simulink model "mcb_pmsm_foc_hall_f28379d"  (R2023b)
settings: Solver=FixedStepDiscrete  StartTime=0.0  StopTime=inf  RelTol=1e-3  EnableMultiTasking=on
InitFcn:
  | mcb_pmsm_foc_hall_f28379d_data;
model workspace (MAT data in the model file):
  encoderResolution = 2000
  hallOffset = '0.5'
  indexOffset = 850
  polePairs = '4'
undefined symbols (not defined in the file): dataType, Down, GPTRIP1SEL, GPTRIP2SEL, inverter, PI_params, pmsm, PosCtrlSpeedLimit, PU_System, target, Ts, Ts_motor, Ts_simulink, Ts_speed, TZ1, TZ2, Up
libraries: simulink x20, c280xlib x17, mcbcontrolslib x9, c2837xDlib x7, c2802xlib x7, svdschedulerlib x5, slpidlib x3, mcbpositiondecoderlib x3, mcbhdlpositiondecoderlib x1, svdutilitieslib x1, mcbplantlib x1, autolibpmsmexterior x1
(part 1 of 4)
settings Model: SimulationMode=external  ExtModeTrigDuration=8  Creator=The MathWorks, Inc.  LastModifiedBy=mdp_3
settings SolverCC: AlgebraicLoopSolver=TrustRegion  AutoInsertRateTranBlk=on
settings DataIOCC: LimitDataPoints=on  SaveFormat=Array  SaveOutput=off  SaveTime=off  ReturnWorkspaceOutputs=off
settings OptimizationCC: DefaultUnderspecifiedDataType=single  OptimizeBlockIOStorage=off  BufferReuse=off  ReuseModelBlockBuffer=off  GlobalBufferReuse=off  ExpressionFolding=off  ExpressionDepthLimit=2147483647  LocalBlockOutputs=off  InitFltsAndDblsToZero=on  NoFixptDivByZeroProtection=on  EfficientFloat2IntCast=on  EfficientMapNaN2IntZero=off  LifeSpan=Inf  MaxStackSize=512  OptimizeDataStoreBuffers=off  BusAssignmentInplaceUpdate=off  EfficientTunableParamExpr=on
settings DebuggingCC: ReadBeforeWriteMsg=DisableAll  WriteAfterWriteMsg=DisableAll  WriteAfterReadMsg=DisableAll  CheckSSInitialOutputMsg=off  SignalResolutionControl=TryResolveAllWithWarning  SolverPrmCheckMsg=warning  InheritedTsInSrcMsg=none  MultiTaskDSMMsg=none  MultiTaskCondExecSysMsg=none  TasksWithSamePriorityMsg=none  SigSpecEnsureSampleTimeMsg=none  IntegerOverflowMsg=none  ParameterPrecisionLossMsg=none  FcnCallInpInsideContextMsg=warning  UnconnectedInputMsg=warning  UnconnectedOutputMsg=warning  UnconnectedLineMsg=warning  AllowSymbolicDim=off  StateNameClashWarn=warning  PregeneratedLibrarySubsystemCodeDiagnostic=none  SFUnexpectedBacktrackingDiag=warning  SFNoUnconditionalDefaultTransitionDiag=warning  SFExecutionAtInitializationDiag=none  IntegerSaturationMsg=none  ArithmeticOperatorsInVariantConditions=warning
settings HardwareCC: ProdBitPerChar=16  ProdBitPerInt=16  ProdBitPerPointer=32  ProdBitPerSizeT=32  ProdBitPerPtrDiffT=32  ProdLargestAtomicInteger=Integer  ProdLargestAtomicFloat=None  ProdWordSize=16  ProdLongLongMode=on  ProdHWDeviceType=Texas Instruments->C2000  TargetBitPerChar=16  TargetBitPerInt=16  TargetBitPerPointer=16  TargetLargestAtomicInteger=Integer  TargetIntDivRoundTo=Zero  TargetEndianess=LittleEndian  TargetWordSize=16  TargetHWDeviceType=TI C2000
settings ModelReferenceCC: EnableRefExpFcnMdlSchedulingChecks=on  PropagateSignalLabelsOutOfModel=off
settings SFSimCC: SimUseLocalCustomCode=off  MATLABDynamicMemAlloc=off
settings SFSimCC: SimCustomHeaderCode=|
  | #include "AHIT_Gimbal_Encoder.h"
  | #include "AHIT_RLS_Encoder_Init.h"
settings SFSimCC: SimUserSources=|
  | AHIT_Gimbal_Encoder.c
  | AHIT_RLS_Encoder_Init.c
settings SFSimCC: SimUserIncludeDirs=|
  | ./include_3
  | ./src_3
settings RTWCC: Description=Embedded Coder  SystemTargetFile=ert.tlc  HardwareBoard=TI Delfino F28379D LaunchPad  TemplateMakefile=ert_default_tmf  GenerateReport=on  RTWUseLocalCustomCode=off  RTWUseSimCustomCode=on  Toolchain=Texas Instruments Code Composer Studio (C2000)  IncludeHyperlinkInReport=on  GenerateTraceInfo=on  GenerateTraceReport=on  GenerateTraceReportSl=on  GenerateTraceReportSf=on  GenerateTraceReportEml=on  DLArmComputeVersion=19.05
settings RTWCC: CustomHeaderCode=|
  | #include "AHIT_Gimbal_Encoder.h"
  | #include "AHIT_RLS_Encoder_Init.h"
settings RTWCC: CustomInclude=|
  | ./include_3
  | ./src_3
settings RTWCC: CustomSource=|
  | AHIT_Gimbal_Encoder.c
  | AHIT_RLS_Encoder_Init.c
settings CodeAppCC: IgnoreCustomStorageClasses=off  CustomSymbolStrType=$N$R$M  StateflowObjectComments=on  InternalIdentifier=Classic
settings ERTTargetCC: CodeReplacementLibrary=TI C28x  MultiwordLength=2048  ConvertIfToSwitch=off  SuppressUnreachableDefaultCases=off  MemSecPackage=tic2000demospkg
settings ConfigComp: CovMetricSettings=dw  CovSaveCumulativeToWorkspaceVar=on  CovSaveSingleToWorkspaceVar=on  CovExternalEMLEnable=off  CovSFcnEnable=off

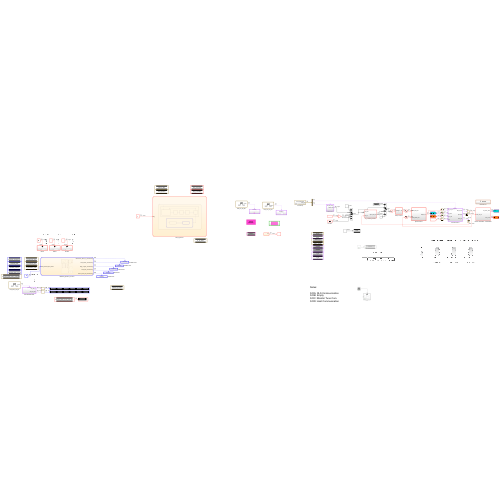
[thumbnail: Simulink's stored preview of the top-level diagram]
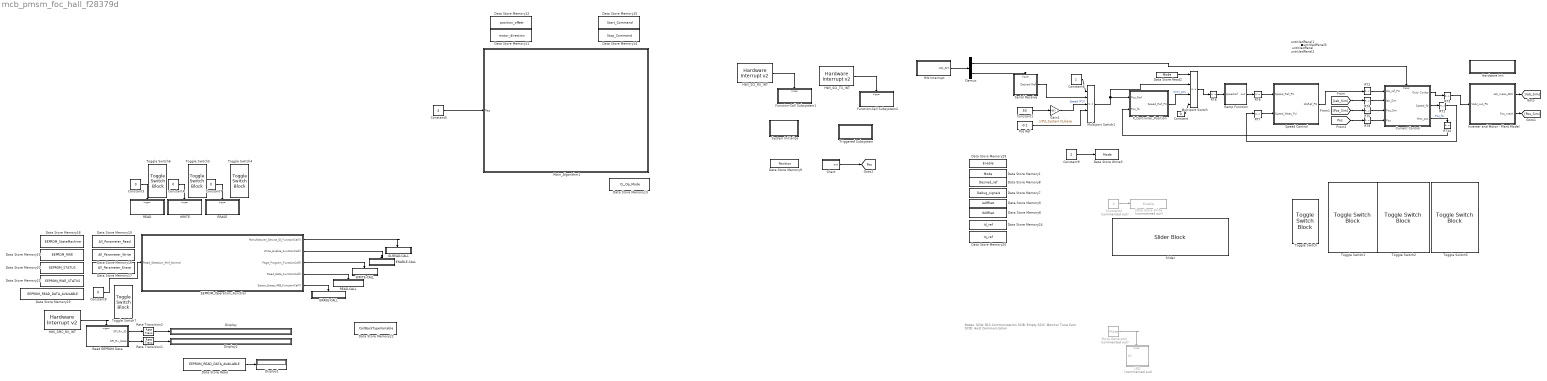
== system mcb_pmsm_foc_hall_f28379d ==
  note: Notes:
      |
      | SCIA: RLS Communication
      | SCIB: Empty
      | SCIC: Monitor Tune Com.
      | SCID: Host Communication
  Chart : Stateflow chart  TreatAsAtomicUnit=on
  Constant : Constant  Value=0  SampleTime=-1
  Constant1 : Constant  Value=50  OutDataTypeStr=single  SampleTime=-1
  Constant2 : Constant  Commented=on  Value=0  OutDataTypeStr=boolean  SampleTime=-1
  Constant3 : Constant  Value=0  OutDataTypeStr=single  SampleTime=-1
  Constant4 : Constant  Value=0  OutDataTypeStr=single  SampleTime=-1
  Constant5 : Constant  Value=4  OutDataTypeStr=uint16  SampleTime=-1
  Constant6 : Constant  SampleTime=-1
  Constant7 : Constant  Value=0  OutDataTypeStr=single  SampleTime=-1
  Constant8 : Constant  Value=0  OutDataTypeStr=boolean  SampleTime=-1
  Constant9 : Constant  Value=2  SampleTime=-1
  Current Control : Subsystem
      settings: RTWSystemCode=Nonreusable function
  Data Store Memory1 : DataStoreMemory  DataStoreName=Mode  ReadBeforeWriteMsg=warning  WriteAfterWriteMsg=warning  WriteAfterReadMsg=warning  InitialValue=500  ShowAdditionalParam=off  OutDataTypeStr=single
  Data Store Memory10 : DataStoreMemory  DataStoreName=All_Parameter_Read  ShowAdditionalParam=off  OutDataTypeStr=boolean
  Data Store Memory11 : DataStoreMemory  DataStoreName=motor_direction  ShowAdditionalParam=off  OutDataTypeStr=uint16
  Data Store Memory12 : DataStoreMemory  DataStoreName=position_offset  ShowAdditionalParam=off  OutDataTypeStr=uint16
  Data Store Memory13 : DataStoreMemory  Description=Closed Loop Operation Mode Selector Variable  DataStoreName=CL_Op_Mode  ShowAdditionalParam=off  OutDataTypeStr=uint16
  Data Store Memory14 : DataStoreMemory  DataStoreName=Stop_Command  ShowAdditionalParam=off  OutDataTypeStr=uint16
  Data Store Memory15 : DataStoreMemory  DataStoreName=Start_Command  ShowAdditionalParam=off  OutDataTypeStr=uint16
  Data Store Memory16 : DataStoreMemory  DataStoreName=All_Parameter_Write  ShowAdditionalParam=off  OutDataTypeStr=boolean
  Data Store Memory17 : DataStoreMemory  DataStoreName=All_Parameter_Erase  ShowAdditionalParam=off  OutDataTypeStr=boolean
  Data Store Memory18 : DataStoreMemory  DataStoreName=EEPROM_StateMachine  InitialValue=t_EEPROM_StateMachine_e.EEPROM_OPERATION_DUMMY_STATE  ShowAdditionalParam=off  OutDataTypeStr=Enum: t_EEPROM_StateMachine_e
  Data Store Memory19 : DataStoreMemory  DataStoreName=EEPROM_RWE  InitialValue=t_EEPROM_RWE_e.EEPROM_DUMMY  ShowAdditionalParam=off  OutDataTypeStr=Enum: t_EEPROM_RWE_e
  Data Store Memory20 : DataStoreMemory  DataStoreName=EEPROM_STATUS  InitialValue=t_EEPROM_STATUS_e.EEPROM_STATUS_NOTBUSY  ShowAdditionalParam=off  OutDataTypeStr=Enum: t_EEPROM_STATUS_e
  Data Store Memory21 : DataStoreMemory  DataStoreName=EEPROM_RWE_STATUS  InitialValue=t_EEPROM_RWE_STATUS_e.EEPROM_RWE_STATUS_DUMMY  ShowAdditionalParam=off  OutDataTypeStr=Enum: t_EEPROM_RWE_STATUS_e
  Data Store Memory22 : DataStoreMemory  DataStoreName=CallBackTypeVariable  ShowAdditionalParam=off  OutDataTypeStr=uint16
  Data Store Memory23 : DataStoreMemory  DataStoreName=EEPROM_READ_DATA_AVAILABLE  ShowAdditionalParam=off  OutDataTypeStr=uint16
  Data Store Memory24 : DataStoreMemory  DataStoreName=Id_ref  ReadBeforeWriteMsg=warning  WriteAfterWriteMsg=warning  WriteAfterReadMsg=warning  ShowAdditionalParam=off  OutDataTypeStr=single
  Data Store Memory25 : DataStoreMemory  DataStoreName=Iq_ref  ReadBeforeWriteMsg=warning  WriteAfterWriteMsg=warning  WriteAfterReadMsg=warning  ShowAdditionalParam=off  OutDataTypeStr=single
  Data Store Memory29 : DataStoreMemory  DataStoreName=Enable  ShowAdditionalParam=off  OutDataTypeStr=boolean
  Data Store Memory5 : DataStoreMemory  DataStoreName=IaOffset  InitialValue=inverter.CtSensAOffset  ShowAdditionalParam=off
  Data Store Memory6 : DataStoreMemory  DataStoreName=IbOffset  InitialValue=inverter.CtSensBOffset  ShowAdditionalParam=off
  Data Store Memory7 : DataStoreMemory  DataStoreName=Debug_signals  ReadBeforeWriteMsg=warning  WriteAfterWriteMsg=warning  WriteAfterReadMsg=warning  InitialValue=5  ShowAdditionalParam=off  OutDataTypeStr=uint16
  Data Store Memory8 : DataStoreMemory  DataStoreName=Desired_ref  ReadBeforeWriteMsg=warning  WriteAfterWriteMsg=warning  WriteAfterReadMsg=warning  InitialValue=500  ShowAdditionalParam=off  OutDataTypeStr=dataType
  Data Store Memory9 : DataStoreMemory  DataStoreName=Position  WriteAfterWriteMsg=warning  ShowAdditionalParam=off  OutDataTypeStr=single
  Data Store Read : DataStoreRead  DataStoreName=EEPROM_READ_DATA_AVAILABLE  IndexOptions=Index vector (dialog)  Indices=1  OutputSizes=1
  Data Store Write : DataStoreWrite  Commented=on  DataStoreName=Enable  IndexOptions=Index vector (dialog)  Indices=1  OutputSizes=1
  Data Store Write3 : DataStoreWrite  DataStoreName=Mode  IndexOptions=Index vector (dialog)  Indices=1  OutputSizes=1
  Data Store Read2 : DataStoreRead  DataStoreName=Mode  IndexOptions=Index vector (dialog)  Indices=1  OutputSizes=1
  Demux : Demux  Outputs=2
  Display : Display
      settings: Format=hex (Stored Integer)
  Display1 : Display
  Display2 : Display
      settings: Format=hex (Stored Integer)
  EEPROM_Operation_Function : Stateflow chart  TreatAsAtomicUnit=on  SystemSampleTime=1/10
  ENABLE-CALL : Subsystem  TreatAsAtomicUnit=on
  ERASE : Subsystem  TreatAsAtomicUnit=on
  ERASE-CALL : Subsystem  TreatAsAtomicUnit=on
  Function-Call Subsystem1 : Subsystem  TreatAsAtomicUnit=on
  Function-Call Subsystem2 : Subsystem  TreatAsAtomicUnit=on
  Gain1 : Gain  Gain=1/PU_System.N_base  RndMeth=Simplest  OutDataTypeStr=Inherit: Same as input
  HW Interrupt : Subsystem  Variant=on  VariantControlMode=sim codegen switching
  HWI_SCI_RX_INT : svdschedulerlib/Hardware Interrupt v2  ISRGroup=ADC - Analog to Digital Converter  ISRName=ADCA1_INT  ISRNumber=32  NumEventsToServe=1  EventsList={'on','EOC event','1';'off','Overflow event','2';'off','Custom event','3'}  SelectedEvents={'event1'}  TaskPriority=25  DisablePreemption=off  ClearInterruptFlagsAtEndOfEvent=on  InterruptDefinitionFile=$(TARGET_ROOT)/registry/interrupts/F2837xS_interrupts.xml  HardwareBoard=F2837x  EnableSimPort=off
      settings: LibrarySourceBlock=c2000lib/Scheduling/Hardware Interrupt
  HWI_SCI_TX_INT : svdschedulerlib/Hardware Interrupt v2  ISRGroup=ADC - Analog to Digital Converter  ISRName=ADCA1_INT  ISRNumber=32  NumEventsToServe=1  EventsList={'on','EOC event','1';'off','Overflow event','2';'off','Custom event','3'}  SelectedEvents={'event1'}  TaskPriority=25  DisablePreemption=off  ClearInterruptFlagsAtEndOfEvent=on  InterruptDefinitionFile=$(TARGET_ROOT)/registry/interrupts/F2837xS_interrupts.xml  HardwareBoard=F2837x  EnableSimPort=off
      settings: LibrarySourceBlock=c2000lib/Scheduling/Hardware Interrupt
  HWI_SPIC_RX_INT : svdschedulerlib/Hardware Interrupt v2  ISRGroup=ADC - Analog to Digital Converter  ISRName=ADCA1_INT  ISRNumber=32  NumEventsToServe=1  EventsList={'on','EOC event','1';'off','Overflow event','2';'off','Custom event','3'}  SelectedEvents={'event1'}  TaskPriority=50  DisablePreemption=off  ClearInterruptFlagsAtEndOfEvent=on  InterruptDefinitionFile=$(TARGET_ROOT)/registry/interrupts/F2837xS_interrupts.xml  HardwareBoard=F2837x  EnableSimPort=off
      settings: LibrarySourceBlock=c2000lib/Scheduling/Hardware Interrupt
  Hardware Init : Subsystem  TreatAsAtomicUnit=on
  ID-READ-CALL : Subsystem  TreatAsAtomicUnit=on
  Inverter and Motor - Plant Model : Subsystem
  LED : Subsystem  Commented=on
  Main_Algorithm1 : Stateflow chart  TreatAsAtomicUnit=on
  Multiport Switch : MultiPortSwitch  Inputs=2  DataPortForDefault=Additional data port  SaturateOnIntegerOverflow=off  InputSameDT=off
  Multiport Switch1 : MultiPortSwitch  DataPortForDefault=Additional data port  SaturateOnIntegerOverflow=off  InputSameDT=off
  P_Controller_Position : Subsystem
  Pos Ref : Constant  Value=-0.1  OutDataTypeStr=single  SampleTime=-1
  Pulse Generator : DiscretePulseGenerator  Commented=on  PulseType=Time based  Period=0.5  PulseWidth=50
  READ : Subsystem  TreatAsAtomicUnit=on
  READ-CALL : Subsystem  TreatAsAtomicUnit=on
  RT{1,6..8,10} (5 alike) : RateTransition  Deterministic=off  OutPortSampleTime=Ts_speed
  RT{2..5,9} (5 alike) : RateTransition  Deterministic=off
  Ramp Function : Subsystem  TreatAsAtomicUnit=on  SystemSampleTime=Ts_speed
  Rate Transition1 : RateTransition  Deterministic=off  OutPortSampleTime=0.2
  Rate Transition2 : RateTransition  Deterministic=off  OutPortSampleTime=0.2
  Read EEPROM Data : Subsystem
  Serial Receive : Subsystem  SystemSampleTime=1e-3
  Slider : SliderBlock  ScaleMax=300
  Speed Control : Subsystem  TreatAsAtomicUnit=on  SystemSampleTime=Ts_speed
  System Initialize : Subsystem  mask(System Initialize){ShowInLibBrowser=0}
      mask prompts: ShowInLibBrowser "Simulink:masks:CustCodeMaskParam1_MP"
      settings: CopyFcn=cccopyfcn(gcb)  OpenFcn=ccopenfcn('System Initialize Function')
      mask Help: eval('feval(''rtwprivate'',''rtwhelpview'',''rtw_sys_initialize_block'')');
      mask Display: disp('System\nInitialize');
  Toggle Switch{,4..7} (5 alike) : ToggleSwitchBlock
      settings: Values={{'Off', 'On'}, [0 1]}
  Toggle Switch1 : ToggleSwitchBlock  LabelPosition=Bottom
      settings: Values={{'Manual Speed Param En', 'Calculated Speed Param En'}, [0 1]}
  Toggle Switch2 : ToggleSwitchBlock  LabelPosition=Bottom
      settings: Values={{'Manual D Loop Param En', 'Calculated D Loop Param En'}, [0 1]}
  Toggle Switch3 : ToggleSwitchBlock  LabelPosition=Bottom
      settings: Values={{'Manual Q Loop Param En', 'Calculated Q Loop Param En'}, [0 1]}
  Triggered Subsystem : Subsystem  TreatAsAtomicUnit=on  SystemSampleTime=0.01
  WRITE : Subsystem  TreatAsAtomicUnit=on
  WRITE-CALL : Subsystem  TreatAsAtomicUnit=on
  untitledPanel : Subsystem  Tag=HiddenForWebPanel  IsWebBlockPanel=on
  untitledPanel1 : Subsystem  Tag=HiddenForWebPanel  IsWebBlockPanel=on
  untitledPanel2 : Subsystem  Tag=HiddenForWebPanel  IsWebBlockPanel=on
  untitledPanel3 : Subsystem  Tag=HiddenForWebPanel  IsWebBlockPanel=on
  tag scope: Pos=global
  wires:
  RT1/1 -> RT7/1
  [Iab_Sim] -> RT4/1
  Speed Control/1(IdqRef_PU) -> RT2/1
  [Pos_Sim] -> RT5/1
  RT2/1 -> Current Control/1(Idq_ref_PU)
  RT4/1 -> Current Control/2(Iab_Sim)
  RT5/1 -> Current Control/3(Pos_Sim)
  Current Control/1(Duty Cycles) -> RT3/1
  RT3/1 -> Inverter and Motor - Plant Model/1(Vabc_out_PU)
  Inverter and Motor - Plant Model/1(Iab_meas_ADC) -> [Iab_Sim]
  Inverter and Motor - Plant Model/2(Pos_mech) -> [Pos_Sim]
  Current Control/2(Speed_fb) -> RT1/1
  Demux/2 -> Serial Receive/Trigger
  Demux/1 -> Current Control/Trigger
  HW Interrupt/1(HW_INT) -> Demux/1
  RT6/1 -> Speed Control/1(Speed_Ref_PU)
  RT7/1 -> Speed Control/2(Speed_Meas_PU)
  RT8/1 -> Ramp Function/1(speedref)
  Ramp Function/1(out) -> RT6/1
  Constant1/1 -> Gain1/1
  Constant2/1 -> Data Store Write/1
  Pulse Generator/1 -> LED/Trigger
  HWI_SCI_TX_INT/1 -> Function-Call Subsystem2/Trigger
  HWI_SCI_RX_INT/1 -> Function-Call Subsystem1/Trigger
  [Pos] -> RT9/1
  RT9/1 -> Current Control/4(Pos)
  EEPROM_Operation_Function/2(Write_Enable_FunctionCall()) -> ENABLE-CALL/Trigger
  Constant7/1 -> ERASE/Trigger
  Rate Transition1/1 -> Display2/1
  Rate Transition2/1 -> Display/1
  Read EEPROM Data/1(SPI_Rx_ID) -> Rate Transition2/1
  EEPROM_Operation_Function/3(Page_Program_FunctionCall()) -> WRITE-CALL/Trigger
  EEPROM_Operation_Function/5(Sector_Erase_4KB_FunctionCall()) -> ERASE-CALL/Trigger
  Read EEPROM Data/2(SPI_Rx_Data) -> Rate Transition1/1
  EEPROM_Operation_Function/4(Read_Data_FunctionCall()) -> READ-CALL/Trigger
  Constant3/1 -> READ/Trigger
  Constant8/1 -> EEPROM_Operation_Function/1(Read_Selection_Mnf_Normal)
  HWI_SPIC_RX_INT/1 -> Read EEPROM Data/Trigger
  Constant4/1 -> WRITE/Trigger
  EEPROM_Operation_Function/1(Manufacturer_Device_ID_FunctionCall()) -> ID-READ-CALL/Trigger
  Data Store Read/1 -> Display1/1
  Chart/1(out) -> [Pos]
  Constant5/1 -> Main_Algorithm1/1(flag)
  Current Control/3(Mec_pos) -> RT10/1  "Pos_fb"
  RT10/1 -> P_Controller_Position/2(Pos_fb)
  Data Store Read2/1 -> Multiport Switch/1
  P_Controller_Position/1(Speed_Ref_PU) -> Multiport Switch/3  "error_pos"
  Multiport Switch/1 -> RT8/1
  Constant/1 -> Multiport Switch/4
  Multiport Switch1/1 -> Multiport Switch/2, P_Controller_Position/1(Pos_Ref)
  Serial Receive/1(Desired Ref) -> Multiport Switch1/2
  Constant6/1 -> Multiport Switch1/1
  Gain1/1 -> Multiport Switch1/3  "Speed (PU)"
  Pos Ref/1 -> Multiport Switch1/4
  Constant9/1 -> Data Store Write3/1

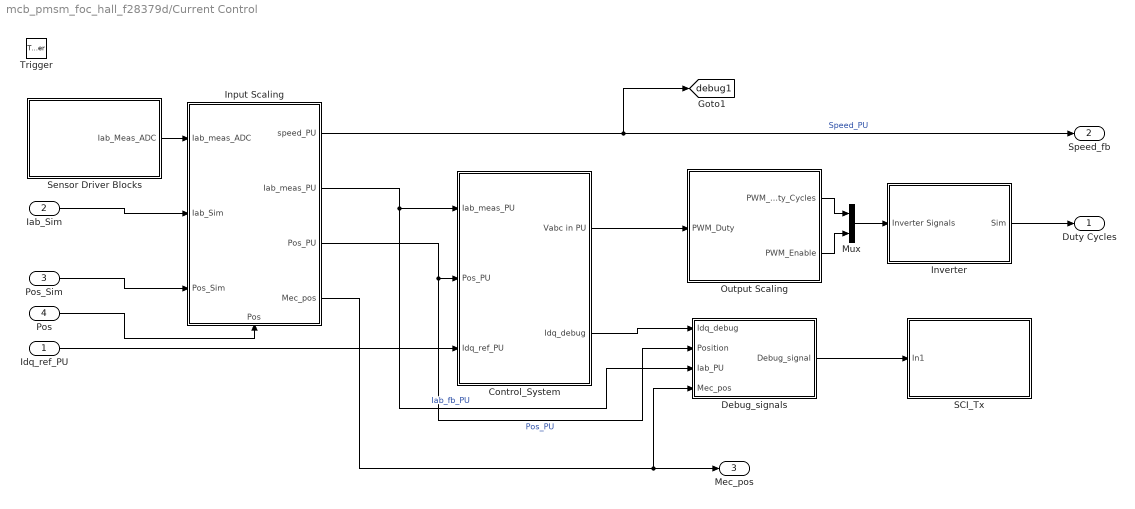
== system mcb_pmsm_foc_hall_f28379d/Current Control ==
  Idq_ref_PU : Inport
  Iab_Sim : Inport  Port=2
  Pos_Sim : Inport  Port=3
  Pos : Inport  Port=4
  Trigger : TriggerPort  TriggerType=function-call  VariantControl=Variant  PortDimensions=1
  Control_System : Subsystem
  Debug_signals : Subsystem
  Input Scaling : Subsystem  Variant=on  VariantControlMode=sim codegen switching  VariantControl=Variant1  PropagateVariantConditions=on
      settings: PortSchema="{\"entries\":[{\"content\":{\"sides\":[{\"content\":{\"connectorIds\":[\"In1\",\"In2\",\"In3\"]},\"type\":\"ConnectorPlacement.EquallySpacedRectSide\",\"uuid\":\"9f2f3667-6d5e-4714-8728-a7ac227716ab\"},{\"content\":{\"connectorIds\":[\"Out1\",\"Out2\",\"Out3\",\"Out4\"],\"side\":\"RIGHT\"},\"type\":\"ConnectorPlacement.EquallySpacedRectSide\",\"uuid\":\"67095e94-5e6f-40af-88f8-fd5db9288dde\"},{\"content\":{\"side\":\"TOP\"},\"type\":\"ConnectorPlacement.EquallySpacedRectSide\",\"uuid\":\"f24a6960-aaac-4f51-bbf1-cf742b655049\"},{\"content\":{\"connectorIds\":[\"In4\"],\"side\":\"BOTTOM\"},\"type\":\"ConnectorPlacement.EquallySpacedRectSide\",\"uuid\":\"f0da2b81-93a9-4692-bf57-8dbb868edb44\"}]},\"type\":\"ConnectorPlacement.EquallySpacedConnector\",\"uuid\":\"0556ef15-0a97-49bd-aca6-6a1187ae6596\"}],\"packageUris\":[\"http://schema.mathworks.com/mf0/Connector/R2020b\"],\"version\":\"1.0\"}"
  Inverter : Subsystem  Variant=on  VariantControlMode=sim codegen switching
  Mux : Mux  Inputs=2
  Output Scaling : Subsystem
  SCI_Tx : Subsystem  Variant=on  VariantControlMode=sim codegen switching
  Sensor Driver Blocks : Subsystem  Variant=on  VariantControlMode=sim codegen switching
  Duty Cycles : Outport  InitialOutput=0  VectorParamsAs1DForOutWhenUnconnected=off
  Speed_fb : Outport  Port=2  InitialOutput=0  VectorParamsAs1DForOutWhenUnconnected=off
  Mec_pos : Outport  Port=3  InitialOutput=0  VectorParamsAs1DForOutWhenUnconnected=off
  tag scope: debug1=global
  wires:
  Control_System/1(Vabc in PU) -> Output Scaling/1(PWM_Duty)
  Input Scaling/3(Pos_PU) -> Debug_signals/2(Position), Control_System/2(Pos_PU)  "Pos_PU"
  Idq_ref_PU/1 -> Control_System/3(Idq_ref_PU)
  Input Scaling/1(speed_PU) -> [debug1], Speed_fb/1  "Speed_PU"
  Input Scaling/2(Iab_meas_PU) -> Debug_signals/3(Iab_PU), Control_System/1(Iab_meas_PU)  "Iab_fb_PU"
  Sensor Driver Blocks/1(Iab_Meas_ADC) -> Input Scaling/1(Iab_meas_ADC)
  Iab_Sim/1 -> Input Scaling/2(Iab_Sim)
  Pos_Sim/1 -> Input Scaling/3(Pos_Sim)
  Inverter/1(Sim) -> Duty Cycles/1
  Debug_signals/1(Debug_signal) -> SCI_Tx/1(In1)
  Mux/1 -> Inverter/1(Inverter Signals)
  Output Scaling/2(PWM_Enable) -> Mux/2
  Output Scaling/1(PWM_Duty_Cycles) -> Mux/1
  Control_System/2(Idq_debug) -> Debug_signals/1(Idq_debug)
  Pos/1 -> Input Scaling/4(Pos)
  Input Scaling/4(Mec_pos) -> Debug_signals/4(Mec_pos), Mec_pos/1

== system mcb_pmsm_foc_hall_f28379d/ENABLE-CALL ==
  function : TriggerPort  TriggerType=function-call  VariantControl=(inherit)
  Chart : Stateflow chart  Commented=on  TreatAsAtomicUnit=on
  Data Store Write1 : DataStoreWrite  DataStoreName=CallBackTypeVariable  IndexOptions=Index vector (dialog)  Indices=1  OutputSizes=1
  Read Command : Constant  Value=6  OutDataTypeStr=uint16  SampleTime=-1
  SPI Transmit : c280xlib/SPI Transmit  Priority=1  SPISelect=SPI_C  ClockPolarity=Rising_edge  ClockPhase=Delay_half_cycle  SPIModule=uint32(0)  Mode=Master  BusSpeed=uint32(1000000)  FirstBitToTransfer=Most significant bit (MSB)  ClockMode=0  BlockFunction=Write  EnableRegisterAddress=on  RegisterAddress=0  OutputDataType=int8  OutputDataLength=1  BlockingMode=on  DataBits=8  UseCustomSSPin=Explicit GPIO calls  ActiveLowSSPin=Active low  Pin=49
  Scope : Scope  Commented=on
  commad : Constant  Value=2  OutDataTypeStr=uint16  SampleTime=-1
  wires:
  Chart/1(output) -> Scope/1
  commad/1 -> Data Store Write1/1
  Read Command/1 -> SPI Transmit/1

== system mcb_pmsm_foc_hall_f28379d/ERASE ==
  Trigger : TriggerPort  VariantControl=(inherit)
  Constant : Constant  OutDataTypeStr=boolean  SampleTime=-1
  Data Store Write2 : DataStoreWrite  DataStoreName=All_Parameter_Erase  IndexOptions=Index vector (dialog)  Indices=1  OutputSizes=1
  wires:
  Constant/1 -> Data Store Write2/1

== system mcb_pmsm_foc_hall_f28379d/ERASE-CALL ==
  function : TriggerPort  TriggerType=function-call  VariantControl=(inherit)
  Chart : Stateflow chart  Commented=on  TreatAsAtomicUnit=on
  Constant : Constant  Value=zeros(3,1)  OutDataTypeStr=uint16  SampleTime=-1
  Data Store Write1 : DataStoreWrite  DataStoreName=CallBackTypeVariable  IndexOptions=Index vector (dialog)  Indices=1  OutputSizes=1
  Mux : Mux  Inputs=2
  Read Command : Constant  Value=32  OutDataTypeStr=uint16  SampleTime=-1
  SPI Transmit : c280xlib/SPI Transmit  Priority=1  SPISelect=SPI_C  ClockPolarity=Rising_edge  ClockPhase=Delay_half_cycle  SPIModule=uint32(0)  Mode=Master  BusSpeed=uint32(1000000)  FirstBitToTransfer=Most significant bit (MSB)  ClockMode=0  BlockFunction=Write  EnableRegisterAddress=on  RegisterAddress=0  OutputDataType=int8  OutputDataLength=1  BlockingMode=on  DataBits=8  UseCustomSSPin=Explicit GPIO calls  ActiveLowSSPin=Active low  Pin=49
  Scope : Scope  Commented=on
  commad : Constant  Value=5  OutDataTypeStr=uint16  SampleTime=-1
  wires:
  Chart/1(output) -> Scope/1
  commad/1 -> Data Store Write1/1
  Constant/1 -> Mux/2  "SPI_Tx_Dummy1"
  Read Command/1 -> Mux/1
  Mux/1 -> SPI Transmit/1  "TX_DATA"

== system mcb_pmsm_foc_hall_f28379d/Function-Call Subsystem1 ==
  function : TriggerPort  TriggerType=function-call  VariantControl=(inherit)
  Data Type Conversion : DataTypeConversion  OutDataTypeStr=uint16  SaturateOnIntegerOverflow=off  RndMeth=Floor
  SCI Receive : c280xlib/SCI Receive  Priority=2  sciModule=A  dataHead=''  headerCheckMaxCount=0  dataTail=''  dataType=uint8  dataLenOptions=Length via dialog  dataDim=1  maxDataLength=1  initValue=0  errOption=Output the last received value  errValue=0  sampleTime=-1  blockingMode=off  timeOut=inf  outputStatus=off
      settings: LibrarySourceBlock=c2837xDlib/SCI Receive
  System Update : Subsystem  mask(System Update){ShowInLibBrowser=0}
      mask prompts: ShowInLibBrowser "Simulink:masks:CustCodeMaskParam1_MP"
      settings: CopyFcn=cccopyfcn(gcb)  OpenFcn=ccopenfcn('System Update Function')
      mask Help: eval('feval(''rtwprivate'',''rtwhelpview'',''rtw_sys_update_block'')');
      mask Display: disp('System\nUpdate');
  Terminator : Terminator
  wires:
  SCI Receive/1 -> Data Type Conversion/1
  Data Type Conversion/1 -> Terminator/1

== system mcb_pmsm_foc_hall_f28379d/Function-Call Subsystem2 ==
  function : TriggerPort  TriggerType=function-call  VariantControl=(inherit)
  SCI Transmit : c280xlib/SCI Transmit  sciModule=A  dataHead=''  dataTail=''  frameSize=1  blockingMode=off  outputStatus=off
      settings: LibrarySourceBlock=c2837xDlib/SCI Transmit

== system mcb_pmsm_foc_hall_f28379d/HW Interrupt ==
  Code Generation : Subsystem  VariantControl=(codegen)
  Simulation : Subsystem  VariantControl=(sim)
  HW_INT : Outport  VectorParamsAs1DForOutWhenUnconnected=off  OutputFunctionCall=on

== system mcb_pmsm_foc_hall_f28379d/Hardware Init ==
  note: Power UP Regulator
  6PWM_Mode : Constant  Priority=1000  Commented=on  Value=0x3A16  OutDataTypeStr=uint16  SampleTime=-1
  ADC_Gain_Setting : Constant  Priority=1000  Commented=on  Value=inverter.SPI_Gain_Setting  OutDataTypeStr=uint16  SampleTime=-1
  Constant : Constant  OutDataTypeStr=boolean  SampleTime=-1
  Constant1 : Constant  OutDataTypeStr=boolean  SampleTime=-1
  Constant2 : Constant  OutDataTypeStr=boolean  SampleTime=-1
  Digital Output : c2837xDlib/Digital Output  GPIO_Number=GPIO144~GPIO151  GPIO_Bit0=off  GPIO_BIT0_Toggle=off  GPIO_Bit1=on  GPIO_BIT1_Toggle=off  GPIO_Bit2=off  GPIO_BIT2_Toggle=off  GPIO_Bit3=off  GPIO_BIT3_Toggle=off  GPIO_Bit4=off  GPIO_BIT4_Toggle=off  GPIO_Bit5=off  GPIO_BIT5_Toggle=off  GPIO_Bit6=off  GPIO_BIT6_Toggle=off  GPIO_Bit7=off  GPIO_BIT7_Toggle=off
  Digital Output1 : c2837xDlib/Digital Output  GPIO_Number=GPIO144~GPIO151  GPIO_Bit0=off  GPIO_BIT0_Toggle=off  GPIO_Bit1=off  GPIO_BIT1_Toggle=off  GPIO_Bit2=on  GPIO_BIT2_Toggle=off  GPIO_Bit3=off  GPIO_BIT3_Toggle=off  GPIO_Bit4=off  GPIO_BIT4_Toggle=off  GPIO_Bit5=off  GPIO_BIT5_Toggle=off  GPIO_Bit6=off  GPIO_BIT6_Toggle=off  GPIO_Bit7=off  GPIO_BIT7_Toggle=off
  Digital Output2 : c2837xDlib/Digital Output  GPIO_Number=GPIO144~GPIO151  GPIO_Bit0=off  GPIO_BIT0_Toggle=off  GPIO_Bit1=off  GPIO_BIT1_Toggle=off  GPIO_Bit2=off  GPIO_BIT2_Toggle=off  GPIO_Bit3=on  GPIO_BIT3_Toggle=off  GPIO_Bit4=off  GPIO_BIT4_Toggle=off  GPIO_Bit5=off  GPIO_BIT5_Toggle=off  GPIO_Bit6=off  GPIO_BIT6_Toggle=off  GPIO_Bit7=off  GPIO_BIT7_Toggle=off
  Event Listener : EventListener  DisableCoverage=on  EventName=reset
  Mux : Mux  Commented=on  Inputs=2
  Variant Subsystem : Subsystem  Commented=on  Variant=on  VariantControlMode=sim codegen switching
  wires:
  6PWM_Mode/1 -> Mux/1
  ADC_Gain_Setting/1 -> Mux/2
  Mux/1 -> Variant Subsystem/1(In1)
  Constant/1 -> Digital Output/1
  Constant1/1 -> Digital Output1/1
  Constant2/1 -> Digital Output2/1

== system mcb_pmsm_foc_hall_f28379d/ID-READ-CALL ==
  function : TriggerPort  TriggerType=function-call  VariantControl=(inherit)
  Chart : Stateflow chart  Commented=on  TreatAsAtomicUnit=on
  Constant : Constant  Value=zeros(3,1)  OutDataTypeStr=uint16  SampleTime=-1
  Data Store Write1 : DataStoreWrite  DataStoreName=CallBackTypeVariable  IndexOptions=Index vector (dialog)  Indices=1  OutputSizes=1
  Mux : Mux  Inputs=3
  Read Address : Constant  Value=[0 0]  OutDataTypeStr=uint16  SampleTime=-1
  Read Command : Constant  Value=144  OutDataTypeStr=uint16  SampleTime=-1
  SPI Transmit : c280xlib/SPI Transmit  Priority=1  SPISelect=SPI_C  ClockPolarity=Rising_edge  ClockPhase=Delay_half_cycle  SPIModule=uint32(0)  Mode=Master  BusSpeed=uint32(1000000)  FirstBitToTransfer=Most significant bit (MSB)  ClockMode=0  BlockFunction=Write  EnableRegisterAddress=on  RegisterAddress=0  OutputDataType=int8  OutputDataLength=1  BlockingMode=on  DataBits=8  UseCustomSSPin=Explicit GPIO calls  ActiveLowSSPin=Active low  Pin=49
  Scope : Scope  Commented=on
  commad : Constant  OutDataTypeStr=uint16  SampleTime=-1
  wires:
  Chart/1(output) -> Scope/1
  Read Address/1 -> Mux/2
  Read Command/1 -> Mux/1
  Constant/1 -> Mux/3  "SPI_Tx_Dummy1"
  Mux/1 -> SPI Transmit/1  "TX_DATA"
  commad/1 -> Data Store Write1/1

== system mcb_pmsm_foc_hall_f28379d/Inverter and Motor - Plant Model ==
  Vabc_out_PU : Inport
  Codegeneration : Subsystem
  Simulation : Subsystem
  Variant Sink : VariantSink  VariantControlMode=sim codegen switching
  Variant Source : VariantSource  VariantControlMode=sim codegen switching
  Variant Source1 : VariantSource  VariantControlMode=sim codegen switching
  Iab_meas_ADC : Outport  VectorParamsAs1DForOutWhenUnconnected=off
  Pos_mech : Outport  Port=2  VectorParamsAs1DForOutWhenUnconnected=off
  wires:
  Codegeneration/2(Pos_fb_Sim) -> Variant Source1/1
  Codegeneration/1(Iab_fb_Sim) -> Variant Source/1
  Variant Source1/1 -> Pos_mech/1
  Variant Sink/1 -> Codegeneration/1(Duty_Cycles)
  Variant Source/1 -> Iab_meas_ADC/1
  Simulation/1(Iab_fb_Sim) -> Variant Source/2
  Variant Sink/2 -> Simulation/1(Duty_Cycles)
  Simulation/2(Pos_fb_Sim) -> Variant Source1/2
  Vabc_out_PU/1 -> Variant Sink/1

== system mcb_pmsm_foc_hall_f28379d/LED ==
  In1 : Inport
  Trigger : TriggerPort  VariantControl=(inherit)  PortDimensions=1
  Constant : Constant  OutDataTypeStr=boolean
  Constant1 : Constant  OutDataTypeStr=boolean
  Digital Output : c2837xDlib/Digital Output  GPIO_Number=GPIO120~GPIO127  GPIO_Bit0=off  GPIO_BIT0_Toggle=off  GPIO_Bit1=off  GPIO_BIT1_Toggle=off  GPIO_Bit2=off  GPIO_BIT2_Toggle=off  GPIO_Bit3=off  GPIO_BIT3_Toggle=off  GPIO_Bit4=off  GPIO_BIT4_Toggle=off  GPIO_Bit5=off  GPIO_BIT5_Toggle=off  GPIO_Bit6=off  GPIO_BIT6_Toggle=off  GPIO_Bit7=on  GPIO_BIT7_Toggle=on
  Digital Output1 : c2837xDlib/Digital Output  GPIO_Number=GPIO128~GPIO135  GPIO_Bit0=on  GPIO_BIT0_Toggle=on  GPIO_Bit1=off  GPIO_BIT1_Toggle=off  GPIO_Bit2=off  GPIO_BIT2_Toggle=off  GPIO_Bit3=off  GPIO_BIT3_Toggle=off  GPIO_Bit4=off  GPIO_BIT4_Toggle=off  GPIO_Bit5=off  GPIO_BIT5_Toggle=off  GPIO_Bit6=off  GPIO_BIT6_Toggle=off  GPIO_Bit7=off  GPIO_BIT7_Toggle=off
  wires:
  Constant1/1 -> Digital Output1/1
  Constant/1 -> Digital Output/1

== system mcb_pmsm_foc_hall_f28379d/P_Controller_Position ==
  Pos_Ref : Inport
  Pos_fb : Inport  Port=2
  Constant : Constant  Value=0.01  OutDataTypeStr=dataType  SampleTime=-1
  Divide : Product  Inputs=**  OutDataTypeStr=dataType  RndMeth=Simplest
  Saturation : Saturate  UpperLimit=PosCtrlSpeedLimit  LowerLimit=-PosCtrlSpeedLimit
  Sum : Sum  Inputs=|+-  OutDataTypeStr=Inherit: Same as first input
  Speed_Ref_PU : Outport
  wires:
  Constant/1 -> Divide/2
  Saturation/1 -> Speed_Ref_PU/1
  Divide/1 -> Saturation/1
  Pos_Ref/1 -> Sum/1
  Pos_fb/1 -> Sum/2
  Sum/1 -> Divide/1

== system mcb_pmsm_foc_hall_f28379d/READ ==
  Trigger : TriggerPort  VariantControl=(inherit)
  Constant : Constant  OutDataTypeStr=boolean  SampleTime=-1
  Data Store Write1 : DataStoreWrite  DataStoreName=All_Parameter_Read  IndexOptions=Index vector (dialog)  Indices=1  OutputSizes=1
  wires:
  Constant/1 -> Data Store Write1/1

== system mcb_pmsm_foc_hall_f28379d/READ-CALL ==
  function : TriggerPort  TriggerType=function-call  VariantControl=(inherit)
  Chart : Stateflow chart  Commented=on  TreatAsAtomicUnit=on
  Constant : Constant  Value=[0 0]  OutDataTypeStr=uint16  SampleTime=-1
  Data Store Write1 : DataStoreWrite  DataStoreName=CallBackTypeVariable  IndexOptions=Index vector (dialog)  Indices=1  OutputSizes=1
  Mux : Mux  Inputs=3
  Read Address : Constant  Value=[0 0 0]  OutDataTypeStr=uint16  SampleTime=-1
  Read Command : Constant  Value=3  OutDataTypeStr=uint16  SampleTime=-1
  SPI Transmit : c280xlib/SPI Transmit  Priority=1  SPISelect=SPI_C  ClockPolarity=Rising_edge  ClockPhase=Delay_half_cycle  SPIModule=uint32(0)  Mode=Master  BusSpeed=uint32(1000000)  FirstBitToTransfer=Most significant bit (MSB)  ClockMode=0  BlockFunction=Write  EnableRegisterAddress=on  RegisterAddress=0  OutputDataType=int8  OutputDataLength=1  BlockingMode=on  DataBits=8  UseCustomSSPin=Explicit GPIO calls  ActiveLowSSPin=Active low  Pin=49
  Scope : Scope  Commented=on
  commad : Constant  Value=4  OutDataTypeStr=uint16  SampleTime=-1
  wires:
  Chart/1(output) -> Scope/1
  commad/1 -> Data Store Write1/1
  Mux/1 -> SPI Transmit/1  "TX_DATA"
  Read Address/1 -> Mux/2
  Constant/1 -> Mux/3  "SPI_Tx_Dummy1"
  Read Command/1 -> Mux/1

== system mcb_pmsm_foc_hall_f28379d/Ramp Function ==
  speedref : Inport
  Chart : Stateflow chart  TreatAsAtomicUnit=on
  Constant : Constant  Value=0.1  OutDataTypeStr=single  SampleTime=-1
  Constant1 : Constant  Value=0.1  OutDataTypeStr=single  SampleTime=-1
  Constant2 : Constant  Value=Ts_speed  OutDataTypeStr=single  SampleTime=-1
  out : Outport
  wires:
  Constant1/1 -> Chart/3(speedDeceleration)
  Constant2/1 -> Chart/4(slope)
  Constant/1 -> Chart/2(speedAcceleration)
  Chart/1(speed) -> out/1  "out"
  speedref/1 -> Chart/1(speedref)

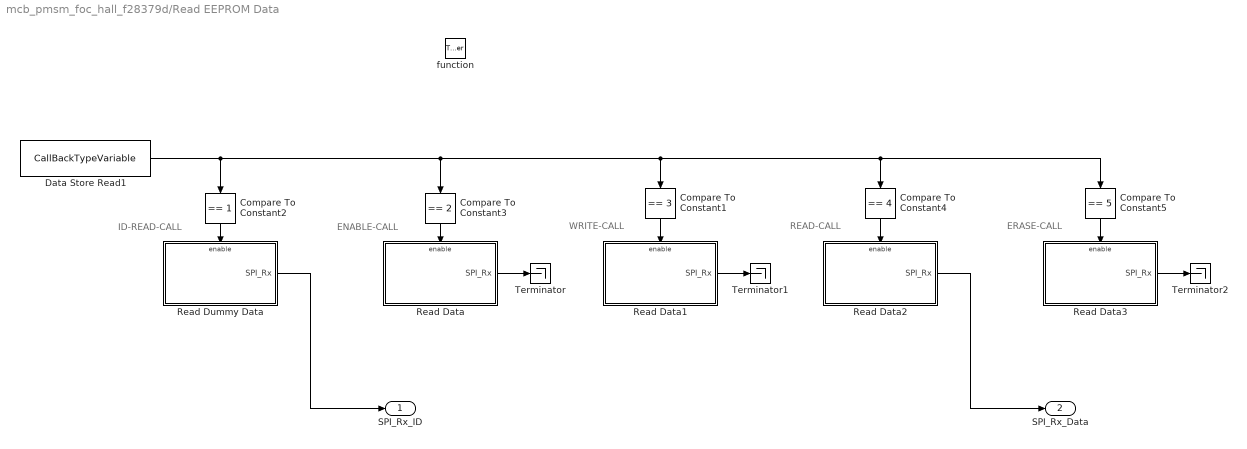
== system mcb_pmsm_foc_hall_f28379d/Read EEPROM Data ==
  note: ID-READ-CALL
  note: WRITE-CALL
  note: READ-CALL
  note: ERASE-CALL
  note: ENABLE-CALL
  function : TriggerPort  TriggerType=function-call  VariantControl=Variant
  Compare To Constant1 : simulink/Logic and Bit Operations/Compare To Constant  relop===  const=3  OutDataTypeStr=boolean  ZeroCross=off
  Compare To Constant2 : simulink/Logic and Bit Operations/Compare To Constant  relop===  const=1  OutDataTypeStr=boolean  ZeroCross=off
  Compare To Constant3 : simulink/Logic and Bit Operations/Compare To Constant  relop===  const=2  OutDataTypeStr=boolean  ZeroCross=off
  Compare To Constant4 : simulink/Logic and Bit Operations/Compare To Constant  relop===  const=4  OutDataTypeStr=boolean  ZeroCross=off
  Compare To Constant5 : simulink/Logic and Bit Operations/Compare To Constant  relop===  const=5  OutDataTypeStr=boolean  ZeroCross=off
  Data Store Read1 : DataStoreRead  DataStoreName=CallBackTypeVariable  IndexOptions=Index vector (dialog)  Indices=1  OutputSizes=1
  Read Data : Subsystem
  Read Data1 : Subsystem
  Read Data2 : Subsystem
  Read Data3 : Subsystem
  Read Dummy Data : Subsystem
  Terminator : Terminator
  Terminator1 : Terminator
  Terminator2 : Terminator
  SPI_Rx_ID : Outport  VectorParamsAs1DForOutWhenUnconnected=off
  SPI_Rx_Data : Outport  Port=2  VectorParamsAs1DForOutWhenUnconnected=off
  wires:
  Compare To Constant3/1 -> Read Data/Enable
  Compare To Constant2/1 -> Read Dummy Data/Enable
  Read Data/1(SPI_Rx) -> Terminator/1
  Read Dummy Data/1(SPI_Rx) -> SPI_Rx_ID/1
  Compare To Constant1/1 -> Read Data1/Enable
  Compare To Constant4/1 -> Read Data2/Enable
  Compare To Constant5/1 -> Read Data3/Enable
  Data Store Read1/1 -> Compare To Constant2/1, Compare To Constant3/1, Compare To Constant1/1, Compare To Constant4/1, Compare To Constant5/1
  Read Data1/1(SPI_Rx) -> Terminator1/1
  Read Data2/1(SPI_Rx) -> SPI_Rx_Data/1
  Read Data3/1(SPI_Rx) -> Terminator2/1

== system mcb_pmsm_foc_hall_f28379d/Serial Receive ==
  SCI_Rx_INT : TriggerPort  TriggerType=function-call  VariantControl=Variant
  Data Store Write : DataStoreWrite  DataStoreName=Enable  IndexOptions=Index vector (dialog)  Indices=1  OutputSizes=1
  Data Store Write1 : DataStoreWrite  DataStoreName=Desired_ref  IndexOptions=Index vector (dialog)  Indices=1  OutputSizes=1
  Data Store Write2 : DataStoreWrite  DataStoreName=Debug_signals  IndexOptions=Index vector (dialog)  Indices=1  OutputSizes=1
  Data Store Write3 : DataStoreWrite  DataStoreName=Mode  IndexOptions=Index vector (dialog)  Indices=1  OutputSizes=1
  Data Type Conversion : DataTypeConversion  OutDataTypeStr=single  SaturateOnIntegerOverflow=off  RndMeth=Floor
  Data_Conditioning_Rx : Subsystem  Variant=on
  SCI_Rx : Subsystem  Variant=on  VariantControlMode=sim codegen switching
  unParse : Subsystem
  Desired Ref : Outport  VectorParamsAs1DForOutWhenUnconnected=off
  wires:
  unParse/2(Debug_signals) -> Data Store Write2/1
  SCI_Rx/1(Data) -> Data_Conditioning_Rx/1(In1)
  unParse/1(Enable_PWM) -> Data Store Write/1
  Data_Conditioning_Rx/1(Desired Ref) -> Desired Ref/1, Data Store Write1/1
  Data_Conditioning_Rx/2(Data) -> unParse/1(Data)
  unParse/3("Selected Referance ") -> Data Type Conversion/1
  Data Type Conversion/1 -> Data Store Write3/1

== system mcb_pmsm_foc_hall_f28379d/Speed Control ==
  Speed_Ref_PU : Inport
  Speed_Meas_PU : Inport  Port=2
  Id_ref : Constant  Value=0  OutDataTypeStr=dataType  SampleTime=Ts_speed
  Mux1 : Mux  Inputs=2
  PI_Controller_Speed : Subsystem
  Speed_Ref_Selector : Subsystem
  IdqRef_PU : Outport  VectorParamsAs1DForOutWhenUnconnected=off
  wires:
  Mux1/1 -> IdqRef_PU/1
  Speed_Meas_PU/1 -> PI_Controller_Speed/2(N_fb), Speed_Ref_Selector/2(Speed_Ref_Open)  "Speed_fb"
  Speed_Ref_PU/1 -> Speed_Ref_Selector/1(Speed_Ref_In)
  PI_Controller_Speed/1(Iq_ref) -> Mux1/2
  Id_ref/1 -> Mux1/1
  Speed_Ref_Selector/1(Speed_Ref_PU) -> PI_Controller_Speed/1(N_ref)  "Speed_Ref"

== system mcb_pmsm_foc_hall_f28379d/System Initialize ==

== system mcb_pmsm_foc_hall_f28379d/Triggered Subsystem ==
  System Update : Subsystem  mask(System Update){ShowInLibBrowser=0}
      mask prompts: ShowInLibBrowser "Simulink:masks:CustCodeMaskParam1_MP"
      settings: CopyFcn=cccopyfcn(gcb)  OpenFcn=ccopenfcn('System Update Function')
      mask Help: eval('feval(''rtwprivate'',''rtwhelpview'',''rtw_sys_update_block'')');
      mask Display: disp('System\nUpdate');

== system mcb_pmsm_foc_hall_f28379d/WRITE ==
  Trigger : TriggerPort  VariantControl=(inherit)
  Constant : Constant  OutDataTypeStr=boolean  SampleTime=-1
  Data Store Write1 : DataStoreWrite  DataStoreName=All_Parameter_Write  IndexOptions=Index vector (dialog)  Indices=1  OutputSizes=1
  wires:
  Constant/1 -> Data Store Write1/1

== system mcb_pmsm_foc_hall_f28379d/WRITE-CALL ==
  function : TriggerPort  TriggerType=function-call  VariantControl=(inherit)
  Chart : Stateflow chart  Commented=on  TreatAsAtomicUnit=on
  Data Store Read1 : DataStoreRead  DataStoreName=motor_direction  IndexOptions=Index vector (dialog)  Indices=1  OutputSizes=1
  Data Store Read2 : DataStoreRead  DataStoreName=position_offset  IndexOptions=Index vector (dialog)  Indices=1  OutputSizes=1
  Data Store Write1 : DataStoreWrite  DataStoreName=CallBackTypeVariable  IndexOptions=Index vector (dialog)  Indices=1  OutputSizes=1
  Mux : Mux
  Read Address : Constant  Value=[0 0 0]  OutDataTypeStr=uint16  SampleTime=-1
  Read Command : Constant  Value=2  OutDataTypeStr=uint16  SampleTime=-1
  SPI Transmit : c280xlib/SPI Transmit  Priority=1  SPISelect=SPI_C  ClockPolarity=Rising_edge  ClockPhase=Delay_half_cycle  SPIModule=uint32(0)  Mode=Master  BusSpeed=uint32(1000000)  FirstBitToTransfer=Most significant bit (MSB)  ClockMode=0  BlockFunction=Write  EnableRegisterAddress=on  RegisterAddress=0  OutputDataType=int8  OutputDataLength=1  BlockingMode=on  DataBits=8  UseCustomSSPin=Explicit GPIO calls  ActiveLowSSPin=Active low  Pin=49
  Scope : Scope  Commented=on
  commad : Constant  Value=3  OutDataTypeStr=uint16  SampleTime=-1
  wires:
  Chart/1(output) -> Scope/1
  commad/1 -> Data Store Write1/1
  Read Command/1 -> Mux/1
  Mux/1 -> SPI Transmit/1  "TX_DATA"
  Read Address/1 -> Mux/2
  Data Store Read1/1 -> Mux/3  "SPI_Tx_Dummy1"
  Data Store Read2/1 -> Mux/4  "SPI_Tx_Dummy1"

== system mcb_pmsm_foc_hall_f28379d/untitledPanel ==
  Slider : SliderBlock  Tag=HiddenForWebPanel  PanelInfo="{\"addnFilesFolder\":\"\",\"height\":50,\"includeDebugPackages\":false,\"left\":18,\"outputFolder\":\"\",\"panelId\":\"panelId-13a995d7-367b-4ece-a822-516db81000d9\",\"popoutMode\":\"\",\"standaloneTitle\":\"\",\"top\":18,\"type\":\"panelChild\",\"version\":\"2019b\",\"width\":431,\"zIndex\":1500004}"  ScaleMax=0.3
  Slider1 : SliderBlock  Tag=HiddenForWebPanel  PanelInfo="{\"addnFilesFolder\":\"\",\"height\":63,\"includeDebugPackages\":false,\"left\":18,\"outputFolder\":\"\",\"panelId\":\"panelId-13a995d7-367b-4ece-a822-516db81000d9\",\"popoutMode\":\"\",\"standaloneTitle\":\"\",\"top\":93,\"type\":\"panelChild\",\"version\":\"2019b\",\"width\":431,\"zIndex\":1500002}"  ScaleMax=0.0005
  panelInfo : PanelWebBlock  Tag=HiddenForWebPanel  PanelInfo="{\"addnFilesFolder\":\"\",\"compacted\":false,\"height\":178,\"includeDebugPackages\":false,\"isActiveTab\":true,\"left\":192,\"name\":\"Panel\",\"outputFolder\":\"\",\"panelId\":\"panelId-13a995d7-367b-4ece-a822-516db81000d9\",\"popoutData\":{\"height\":241,\"left\":224,\"maximized\":false,\"top\":460,\"width\":484},\"popoutMode\":\"windowHidden\",\"standaloneTitle\":\"\",\"tabIndex\":0,\"tabbedSetId\":\"tabbedSet0732174381\",\"top\":292,\"type\":\"panel\",\"version\":\"2019b\",\"visible\":true,\"width\":471,\"zIndex\":1500002}"

== system mcb_pmsm_foc_hall_f28379d/untitledPanel1 ==
  Speed Parameter Ki : SliderBlock  Tag=HiddenForWebPanel  PanelInfo="{\"addnFilesFolder\":\"\",\"height\":48,\"includeDebugPackages\":false,\"left\":14,\"outputFolder\":\"\",\"panelId\":\"panelId-88cac932-804f-4600-bfbb-f4f508c556e5\",\"popoutMode\":\"\",\"standaloneTitle\":\"\",\"top\":94,\"type\":\"panelChild\",\"version\":\"2019b\",\"width\":373,\"zIndex\":1500002}"  ScaleMax=0.1
  Speed Parameter Kp : SliderBlock  Tag=HiddenForWebPanel  PanelInfo="{\"addnFilesFolder\":\"\",\"height\":48,\"includeDebugPackages\":false,\"left\":14,\"outputFolder\":\"\",\"panelId\":\"panelId-88cac932-804f-4600-bfbb-f4f508c556e5\",\"popoutMode\":\"\",\"standaloneTitle\":\"\",\"top\":14,\"type\":\"panelChild\",\"version\":\"2019b\",\"width\":373,\"zIndex\":1500004}"  ScaleMax=10
  panelInfo : PanelWebBlock  Tag=HiddenForWebPanel  PanelInfo="{\"addnFilesFolder\":\"\",\"compacted\":true,\"height\":158,\"includeDebugPackages\":false,\"isActiveTab\":true,\"left\":15,\"name\":\"Panel1\",\"outputFolder\":\"\",\"panelId\":\"panelId-88cac932-804f-4600-bfbb-f4f508c556e5\",\"popoutMode\":\"\",\"standaloneTitle\":\"\",\"tabIndex\":0,\"tabbedSetId\":\"tabbedSet0923835679\",\"top\":12,\"type\":\"panel\",\"version\":\"2019b\",\"visible\":true,\"width\":401,\"zIndex\":1500004}"  PanelSnapshot=<binary blob, 12884 chars, not shown>

== system mcb_pmsm_foc_hall_f28379d/untitledPanel2 ==
  Slider : SliderBlock  Tag=HiddenForWebPanel  PanelInfo="{\"addnFilesFolder\":\"\",\"height\":59,\"includeDebugPackages\":false,\"left\":13,\"outputFolder\":\"\",\"panelId\":\"panelId-704216e3-3f83-4780-91a6-1b031308e76c\",\"popoutMode\":\"\",\"standaloneTitle\":\"\",\"top\":13,\"type\":\"panelChild\",\"version\":\"2019b\",\"width\":282,\"zIndex\":1500004}"  ScaleMax=5
  Slider1 : SliderBlock  Tag=HiddenForWebPanel  PanelInfo="{\"addnFilesFolder\":\"\",\"height\":59,\"includeDebugPackages\":false,\"left\":13,\"outputFolder\":\"\",\"panelId\":\"panelId-704216e3-3f83-4780-91a6-1b031308e76c\",\"popoutMode\":\"\",\"standaloneTitle\":\"\",\"top\":79,\"type\":\"panelChild\",\"version\":\"2019b\",\"width\":282,\"zIndex\":1500002}"  ScaleMax=0.5
  panelInfo : PanelWebBlock  Tag=HiddenForWebPanel  PanelInfo="{\"addnFilesFolder\":\"\",\"compacted\":true,\"height\":155,\"includeDebugPackages\":false,\"isActiveTab\":true,\"left\":94,\"name\":\"Panel2\",\"outputFolder\":\"\",\"panelId\":\"panelId-704216e3-3f83-4780-91a6-1b031308e76c\",\"popoutMode\":\"\",\"standaloneTitle\":\"\",\"tabIndex\":0,\"tabbedSetId\":\"tabbedSet4448288332\",\"top\":9,\"type\":\"panel\",\"version\":\"2019b\",\"visible\":true,\"width\":310,\"zIndex\":1500006}"  PanelSnapshot=<binary blob, 11088 chars, not shown>

== system mcb_pmsm_foc_hall_f28379d/untitledPanel3 ==
  Slider : SliderBlock  Tag=HiddenForWebPanel  PanelInfo="{\"addnFilesFolder\":\"\",\"height\":61,\"includeDebugPackages\":false,\"left\":16,\"outputFolder\":\"\",\"panelId\":\"panelId-880ba189-6bb5-44bd-a37f-51b687412f3f\",\"popoutMode\":\"\",\"standaloneTitle\":\"\",\"top\":15,\"type\":\"panelChild\",\"version\":\"2019b\",\"width\":291,\"zIndex\":1500004}"  ScaleMax=5
  Slider1 : SliderBlock  Tag=HiddenForWebPanel  PanelInfo="{\"addnFilesFolder\":\"\",\"height\":61,\"includeDebugPackages\":false,\"left\":16,\"outputFolder\":\"\",\"panelId\":\"panelId-880ba189-6bb5-44bd-a37f-51b687412f3f\",\"popoutMode\":\"\",\"standaloneTitle\":\"\",\"top\":85,\"type\":\"panelChild\",\"version\":\"2019b\",\"width\":291,\"zIndex\":1500002}"  ScaleMax=0.5
  panelInfo : PanelWebBlock  Tag=HiddenForWebPanel  PanelInfo="{\"addnFilesFolder\":\"\",\"compacted\":true,\"height\":165,\"includeDebugPackages\":false,\"isActiveTab\":true,\"left\":162,\"name\":\"Panel3\",\"outputFolder\":\"\",\"panelId\":\"panelId-880ba189-6bb5-44bd-a37f-51b687412f3f\",\"popoutMode\":\"\",\"standaloneTitle\":\"\",\"tabIndex\":0,\"tabbedSetId\":\"tabbedSet4341935357\",\"top\":9,\"type\":\"panel\",\"version\":\"2019b\",\"visible\":true,\"width\":326,\"zIndex\":1500008}"  PanelSnapshot=<binary blob, 11140 chars, not shown>

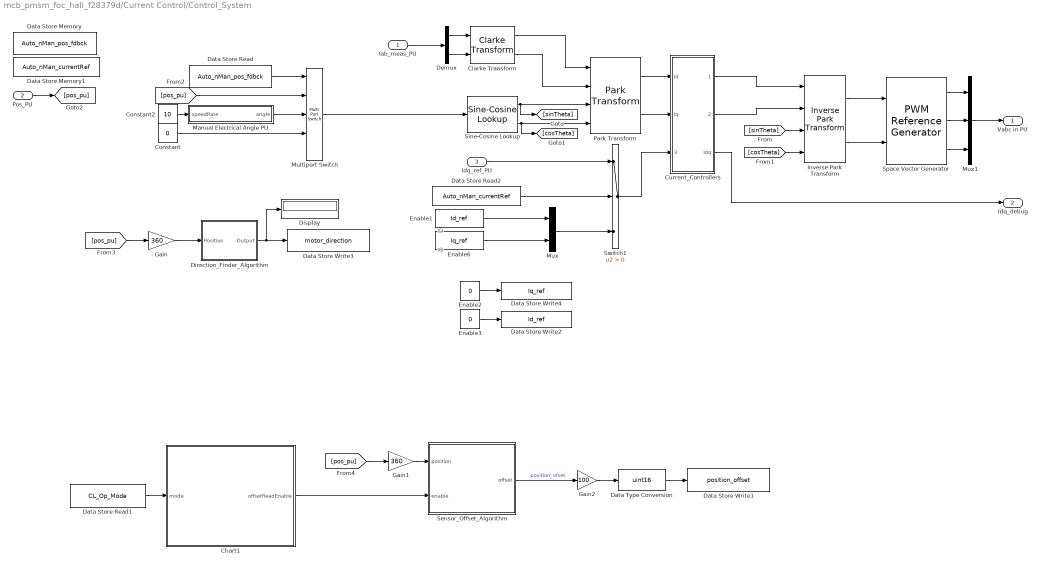
== system mcb_pmsm_foc_hall_f28379d/Current Control/Control_System ==
  note: ID
  note: IQ
  Iab_meas_PU : Inport
  Pos_PU : Inport  Port=2
  Idq_ref_PU : Inport  Port=3
  Chart1 : Stateflow chart  TreatAsAtomicUnit=on
  Clarke Transform : mcbcontrolslib/Clarke Transform  VariantControl=Variant2  PhaseInput=Two inputs  EnPowerInv=off
  Constant : Constant  Value=0  OutDataTypeStr=single  SampleTime=-1
  Constant2 : Constant  Value=10  OutDataTypeStr=single  SampleTime=-1
  Current_Controllers : Subsystem
  Data Store Memory : DataStoreMemory  DataStoreName=Auto_nMan_pos_fdbck  WriteAfterWriteMsg=warning  ShowAdditionalParam=off  OutDataTypeStr=uint16
  Data Store Memory1 : DataStoreMemory  DataStoreName=Auto_nMan_currentRef  WriteAfterWriteMsg=warning  ShowAdditionalParam=off  OutDataTypeStr=boolean
  Data Store Read : DataStoreRead  DataStoreName=Auto_nMan_pos_fdbck  IndexOptions=Index vector (dialog)  Indices=1  OutputSizes=1
  Data Store Read1 : DataStoreRead  DataStoreName=CL_Op_Mode  IndexOptions=Index vector (dialog)  Indices=1  OutputSizes=1
  Data Store Read2 : DataStoreRead  DataStoreName=Auto_nMan_currentRef  IndexOptions=Index vector (dialog)  Indices=1  OutputSizes=1
  Data Store Write1 : DataStoreWrite  DataStoreName=position_offset  IndexOptions=Index vector (dialog)  Indices=1  OutputSizes=1
  Data Store Write2 : DataStoreWrite  DataStoreName=Id_ref  IndexOptions=Index vector (dialog)  Indices=1  OutputSizes=1
  Data Store Write3 : DataStoreWrite  DataStoreName=motor_direction  IndexOptions=Index vector (dialog)  Indices=1  OutputSizes=1
  Data Store Write4 : DataStoreWrite  DataStoreName=Iq_ref  IndexOptions=Index vector (dialog)  Indices=1  OutputSizes=1
  Data Type Conversion : DataTypeConversion  OutDataTypeStr=uint16  SaturateOnIntegerOverflow=off  RndMeth=Floor
  Demux : Demux  Outputs=2
  Direction_Finder_Algorithm : Subsystem
  Display : Display
  Enable1 : DataStoreRead  DataStoreName=Id_ref  IndexOptions=Index vector (dialog)  Indices=1  OutputSizes=1
  Enable2 : Constant  Value=0  OutDataTypeStr=single  SampleTime=-1
  Enable3 : Constant  Value=0  OutDataTypeStr=single  SampleTime=-1
  Enable6 : DataStoreRead  DataStoreName=Iq_ref  IndexOptions=Index vector (dialog)  Indices=1  OutputSizes=1
  Gain : Gain  Gain=360  OutDataTypeStr=single
  Gain1 : Gain  Gain=360  OutDataTypeStr=single
  Gain2 : Gain  Gain=100  OutDataTypeStr=single
  Inverse Park Transform : mcbcontrolslib/Inverse Park Transform  PhaseInput=Two inputs  AxisAlignment=D-axis  ThetaInput=Sine and Cosine electrical position  AngleInput=Per-unit  N_points=1024
  Manual Electrical Angle PU : Stateflow chart  TreatAsAtomicUnit=on
  Multiport Switch : MultiPortSwitch  Inputs=4  SaturateOnIntegerOverflow=off  InputSameDT=off
  Mux : Mux  Inputs=2
  Mux1 : Mux  Inputs=3
  Park Transform : mcbcontrolslib/Park Transform  PhaseInput=Two inputs  AxisAlignment=D-axis  ThetaInput=Sine and Cosine electrical position  AngleInput=Per-unit  N_points=1024
  Sensor_Offset_Algorithm : Stateflow chart  TreatAsAtomicUnit=on
  Sine-Cosine Lookup : mcbcontrolslib/Sine-Cosine Lookup  AngleInput=Per-unit  N_points=1024
  Space Vector Generator : mcbcontrolslib/PWM Reference Generator  inSignal=Valphabeta  modType=SVM: space vector modulation
  Switch1 : Switch  Criteria=u2 > Threshold  OutDataTypeStr=single  SaturateOnIntegerOverflow=off  InputSameDT=off
  Vabc in PU : Outport  VectorParamsAs1DForOutWhenUnconnected=off
  Idq_debug : Outport  Port=2  VectorParamsAs1DForOutWhenUnconnected=off
  wires:
  Mux1/1 -> Vabc in PU/1
  Space Vector Generator/3 -> Mux1/3
  Iab_meas_PU/1 -> Demux/1
  Sine-Cosine Lookup/2 -> Park Transform/4, [cosTheta]
  [cosTheta] -> Inverse Park Transform/4
  Demux/2 -> Clarke Transform/2
  Space Vector Generator/1 -> Mux1/1
  Current_Controllers/1(Vd_ref) -> Inverse Park Transform/1
  Demux/1 -> Clarke Transform/1
  Inverse Park Transform/2 -> Space Vector Generator/2
  Space Vector Generator/2 -> Mux1/2
  Park Transform/2 -> Current_Controllers/2(Iq)
  [sinTheta] -> Inverse Park Transform/3
  Clarke Transform/1 -> Park Transform/1
  Sine-Cosine Lookup/1 -> [sinTheta], Park Transform/3
  Clarke Transform/2 -> Park Transform/2
  Park Transform/1 -> Current_Controllers/1(Id)
  Current_Controllers/2(Vq_ref) -> Inverse Park Transform/2
  Inverse Park Transform/1 -> Space Vector Generator/1
  Current_Controllers/3(Idq) -> Idq_debug/1
  Enable1/1 -> Mux/1
  Enable6/1 -> Mux/2
  Constant2/1 -> Manual Electrical Angle PU/1(speedRate)
  [pos_pu] -> Multiport Switch/2
  Multiport Switch/1 -> Sine-Cosine Lookup/1
  Data Store Read2/1 -> Switch1/2
  Idq_ref_PU/1 -> Switch1/1
  Mux/1 -> Switch1/3
  Switch1/1 -> Current_Controllers/3(Idq_ref_PU)
  Data Store Read1/1 -> Chart1/1(mode)
  Gain/1 -> Direction_Finder_Algorithm/1(Position)
  Direction_Finder_Algorithm/1(Output) -> Display/1, Data Store Write3/1
  Manual Electrical Angle PU/1(angle) -> Multiport Switch/3
  Constant/1 -> Multiport Switch/4
  Data Store Read/1 -> Multiport Switch/1
  Sensor_Offset_Algorithm/1(offset) -> Gain2/1  "position_ofset"
  Chart1/1(offsetReadEnable) -> Sensor_Offset_Algorithm/2(enable)
  Pos_PU/1 -> [pos_pu]
  [pos_pu] -> Gain/1
  [pos_pu] -> Gain1/1
  Gain1/1 -> Sensor_Offset_Algorithm/1(position)
  Gain2/1 -> Data Type Conversion/1
  Data Type Conversion/1 -> Data Store Write1/1
  Enable3/1 -> Data Store Write2/1
  Enable2/1 -> Data Store Write4/1
